simulink model "TwoTank"  (R2020b)
settings: Solver=VariableStepAuto  StartTime=0.0  StopTime=1.5  RelTol=1e-3
settings Model: Creator=Javad  LastModifiedBy=Javad

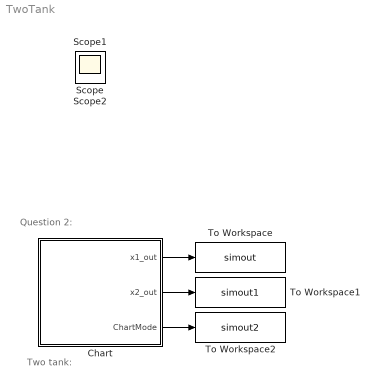
== system TwoTank ==
  note: Two tank:
  note: Question 2:
  Chart : Stateflow chart  TreatAsAtomicUnit=on
  To Workspace : ToWorkspace  VariableName=simout  SaveFormat=Timeseries  SampleTime=-1
  To Workspace1 : ToWorkspace  VariableName=simout1  SaveFormat=Timeseries  SampleTime=-1
  To Workspace2 : ToWorkspace  VariableName=simout2  SaveFormat=Timeseries  SampleTime=-1
  Scope : Scope
  Scope1 : Scope
  Scope2 : Scope
  wires:
  Chart/3(ChartMode) -> To Workspace2/1
  Chart/2(x2_out) -> To Workspace1/1
  Chart/1(x1_out) -> To Workspace/1

== stateflow chart TwoTank/Chart ==
  settings: updateMethod=CONTINUOUS
  state Tank1
    du:
    x1_dot=10-5;
    x2_dot=-7;
    x1_out=x1;
    x2_out=x2;
  state Tank2
    du:
    x1_dot=-5;
    x2_dot=10-7;
    x1_out=x1;
    x2_out=x2;
  (default) -> Tank1 : {x1=3;
      | x2=3;}
  Tank1 -> Tank2 : [x2<=2]{x1=x1;x2=x2;}
  Tank2 -> Tank1 : [x1<=1]{x1=x1;x2=x2;}
  data: x1_out output; x2_out output; x1 local; x2 local; ChartMode output Enum: ChartModeType
  data x1 settings: updateMethod=SF_CONTINUOUS_TIME_DATA
  data x2 settings: updateMethod=SF_CONTINUOUS_TIME_DATA
